simulink model "Main_bikesimulation_old"  (R2022b)
settings: Solver=FixedStepAuto  StartTime=0.0  StopTime=sim_time-0.02  FixedStep=0.001
undefined symbols (not defined in the file): A_d, Ad_t, B_d, Bd_t, bike_model, bike_params, C1, C2, C_t, counter, D1, D2, D_t, e1_max, g, hor_dis, I_balancing_outer, initial_state, initial_state_estimate, k1, k2, Kalman_gain1, Kalman_gain2, linearized_sys, P_balancing_inner, P_balancing_outer, pert_deltadot_state, pert_deltadot_state_fun, pert_phidot_state, pert_phidot_state_fun, Psiref, ref_dis, ref_start_idx, sigbuilder_block, T, Ts, v, Xref, Yref
libraries: simulink x8, slpidlib x2, cstblocks x1, eeGeneralControl x1
(part 2 of 2)

== matlab function Main_bikesimulation_old/Unstable bike model/Track bycicle pose/MATLAB Function ==
  data: Speed input; steer_angle input; beta output; bike_params input; psi_dot output
function [beta, psi_dot] = fcn(Speed, steer_angle, bike_params)
lr       = bike_params(1);
lf       = bike_params(2);
lambda  = bike_params(3);

eff_steering = steer_angle*sin(lambda);

beta = atan(lr /(lr+lf) * tan(eff_steering) );
psi_dot = (Speed / lr) * sin(beta);

== matlab function Main_bikesimulation_old/Sensors/Define true sensor positions on the bike ==
  data: bike_params input; pose input; pose_corrected output
function pose_corrected  = fcn(bike_params, pose)
pose_corrected = pose;

gpsX = bike_params(1); % measured offset of GPS parallel to bike
gpsY = bike_params(2); % measured offset of GPS perpendicular to bike
gpsH = bike_params(3); % measured offset of GPS from ground to GPS

% define pose_l
pose_l = pose;

% Transform to local frame
    pose_l(1) =  pose(1) * cos(pose(3)) + pose(2) * sin(pose(3));
    pose_l(2) = -pose(1) * sin(pose(3)) + pose(2) * cos(pose(3)); 

% define actual positions of GPS 
% pose1 = difference in x in local frame
% pose2 = difference in y in local frame
    pose_l(1) = pose_l(1) + gpsX;
    pose_l(2) = pose_l(2) + gpsY + gpsH*sin(pose(4));

% define actual positions of IMU 


% Transform back to global frame
    pose(1) = pose_l(1) * cos(pose(3)) - pose_l(2) * sin(pose(3));
    pose(2) = pose_l(1) * sin(pose(3)) + pose_l(2) * cos(pose(3));

pose_corrected(1) = pose(1);
pose_corrected(2) = pose(2);

== matlab function Main_bikesimulation_old/Closest point algorithm & Error calculation/Closest point algorithm & Error calculation ==
  settings: updateMethod=DISCRETE  sampleTime=Ts
  data: e1 output; e2 output; dpsiref output; closestpoint_idx output; closestpoint_heading_idx output; Xref_loc input; Yref_loc input; psiref_loc input; X_est input; Y_est input; psi_est input; ref_X output; ref_Y output; ref_psi output; v input
function [e1,e2,dpsiref,closestpoint_idx,closestpoint_heading_idx,ref_X,ref_Y,ref_psi]= fcn(Xref_loc,Yref_loc,psiref_loc,X_est,Y_est,psi_est,v)
%% calculations on a local part of the trajectory

% Each referencepoint has a location (X,Y) and a heading
% The heading is defined in the startup.m file as 'the heading where its coming from' 
% Second point in local reference is current selected closest point
closestpoint_idx=2;

% Search for closest point
% Finding the closest point going forward. Stop searching once next
% distance increases

while (Xref_loc(closestpoint_idx,1)-X_est)^2 + (Yref_loc(closestpoint_idx,1)-Y_est)^2 >= (Xref_loc(closestpoint_idx+1,1)-X_est)^2+(Yref_loc(closestpoint_idx+1,1)-Y_est)^2  && closestpoint_idx <= length(Xref_loc)-2
closestpoint_idx = closestpoint_idx+1;
end

% Select same closest point (for heading error and position error)
closestpoint_heading_idx = closestpoint_idx;


% Calculate X and Y distance from current location to selected closest
% point
dx = X_est - Xref_loc(closestpoint_idx,1);
dy = Y_est - Yref_loc(closestpoint_idx,1);

% Calculate difference in current heading and heading in reference point 
% And limit D_psiref  between -2pi and 2pi
D_psiref=psiref_loc(closestpoint_idx+1,1)-psiref_loc(closestpoint_idx,1);
if D_psiref>=pi
    D_psiref=mod(D_psiref,-2*pi);
end
if D_psiref<=-pi
    D_psiref=mod(D_psiref,2*pi);
end
%IMPROVEMENT: implement an interpolation algoritm
% Calculate distence between point before closest point and current location
dist_true_previous = sqrt((Xref_loc(closestpoint_idx-1,1)-X_est)^2+(Yref_loc(closestpoint_idx-1,1)-Y_est)^2);
% Angle of line between previous closest point and current location
alpha_star = atan((Yref_loc(closestpoint_idx-1,1)-Y_est)/(Xref_loc(closestpoint_idx-1,1)-X_est));
% heading previous closest point - alpha star
alpha_projected_dist = alpha_star-psiref_loc(closestpoint_idx,1);
% the distance from the previous closest point to the projection of the bike on the trajectory
Projected_dist = abs(dist_true_previous*cos(alpha_projected_dist));

compared_dist = sqrt((Xref_loc(closestpoint_idx,1)-Xref_loc(closestpoint_idx-1,1))^2+(Yref_loc(closestpoint_idx,1)-Yref_loc(closestpoint_idx-1,1))^2);

% If bike passes closest point, the heading of the next point will be taken
if Projected_dist >= compared_dist
closestpoint_heading_idx = closestpoint_idx+1;
end

%calculate e1 and e2        
e1= dy*cos(psiref_loc(closestpoint_heading_idx,1)) - dx*sin(psiref_loc(closestpoint_heading_idx,1)); % this make e1 include "direction" automatically
e2= psi_est-psiref_loc(closestpoint_heading_idx,1); %calculate e2

% closest point on the local trajectory
ref_X=Xref_loc(closestpoint_idx,1);
ref_Y=Yref_loc(closestpoint_idx,1);
ref_psi=psiref_loc(closestpoint_heading_idx,1);

 % keep heading error should be between -pi 2 pi
e2 = wrapToPi(e2);
%e2=mod(e2+pi,2*pi)-pi;     

%calculate the time between psiref(idx,1) and psiref(idx+1,1)
dX=Xref_loc(closestpoint_idx+1,1)-ref_X;
dY=Yref_loc(closestpoint_idx+1,1)-ref_Y;
dis=sqrt(dX^2+dY^2);
Ts_psi=dis/v;

% Sample dpsiref
dpsiref=(D_psiref)/Ts_psi;

% Reset closest point index as feedback for local frame selection
closestpoint_idx = closestpoint_idx-1;

end

== matlab function Main_bikesimulation_old/convert steer angle into ref roll/Convert steer angle to roll ==
  data: steer_angle_ref input; roll_ref output; bike_params input; v input
function roll_ref = fcn(steer_angle_ref, bike_params, v)

lambda = bike_params(1);
lr      = bike_params(2);
lf      = bike_params(3);
g      = bike_params(4);

eff_steer_angle = steer_angle_ref*sin(lambda);
roll_ref = -1*atan((tan(eff_steer_angle)*(v^2/(lr+lf)))/g);
